simulink model "playback_data_4"  (R2015a)
settings: Solver=FixedStepDiscrete  SolverMode=SingleTasking  StartTime=0  StopTime=time_recorded(end)  FixedStep=sample_time  RelTol=1e-3
undefined symbols (not defined in the file): A1_notch_f1, A2_notch_f1, A_kalman_transverse, A_kalman_vertical, A_lpf_dtau, A_lpf_fourbar_angles, A_lpf_imu, A_lpf_lateral_angle, A_lpf_leg_spring, B1_lpf_dtau, B1_lpf_fourbar_angles, B1_lpf_imu, B1_lpf_lateral_angle, B1_lpf_leg_spring, B1_notch_f1, B2_lpf_dtau, B2_lpf_fourbar_angles, B2_lpf_imu, B2_lpf_lateral_angle, B2_lpf_leg_spring, B2_notch_f1, B_dx_versus_x0, B_kalman_transverse, B_kalman_vertical, backwards_K_front_of_t_row1, backwards_K_front_of_t_row2, backwards_K_sag_of_t, backwards_P_front_of_t, backwards_P_sag_of_t, C_kalman_transverse, C_kalman_vertical, com_leg_motor, com_torso, contact_threshold, control_start_time, d_ankle_to_foot, d_vertical_com, desired_com_forward_velocity, desired_com_lateral_velocity, desired_initial_leg_roll_left, desired_initial_leg_roll_right, desired_lateral_symmetry_angle, desired_standing_torso_pitch, desired_standing_torso_roll, desired_standing_z, desired_torso_pitch, desired_torso_roll, Discrete, fcut_contact, forward_dx_of_dxstar, forward_x_of_dxstar, g, gain_nodes_sea_torque, HIP_MTR_MAX_CONT_TORQUE, HIP_MTR_MAX_TORQUE, i_leg_motor, i_robot, i_torso, initial_dx_estimate, initial_dy_estimate ... (+75)
libraries: simulink x12, ctrlSharedLib x3
(part 1 of 5)
settings Model: CovSFcnEnable=off  Creator=wmartin  LastModifiedBy=wmartin
settings SolverCC: EnableConcurrentExecution=on
settings DataIOCC: LimitDataPoints=off  MaxDataPoints=1000000000  SaveFormat=StructureWithTime  SignalLogging=off  DSMLogging=off  VisualizeSimOutput=off
settings OptimizationCC: BlockReduction=off  OptimizeBlockIOStorage=off  BufferReuse=off  GlobalBufferReuse=off  ExpressionFolding=off  ExpressionDepthLimit=2147483647  LocalBlockOutputs=off  SimCompilerOptimization=on
settings DebuggingCC: UnderspecifiedInitializationDetection=Classic  MergeDetectMultiDrivingBlocksExec=none  SolverPrmCheckMsg=warning  StateNameClashWarn=warning
settings HardwareCC: ProdIntDivRoundTo=Zero  ProdEndianess=LittleEndian  ProdLongLongMode=on  ProdHWDeviceType=Generic->32-bit x86 compatible
settings ModelReferenceCC: UpdateModelReferenceTargets=IfOutOfDate  ModelReferenceNumInstancesAllowed=Single  ModelReferenceMinAlgLoopOccurrences=on
settings RTWCC: SystemTargetFile=slrt.tlc  TemplateMakefile=slrt_default_tmf  Description=Simulink Real-Time  RTWVerbose=off  RTWCompilerOptimization=on
settings CodeAppCC: MaxIdLength=256
settings SimulinkRealTimeCC: GeneratePreprocessorConditionals=Disable all

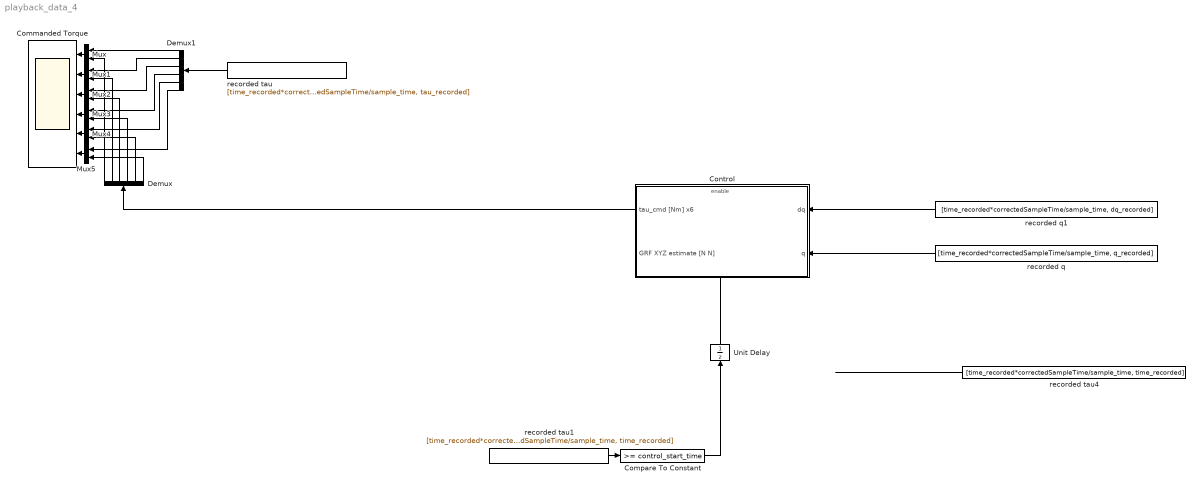
== system playback_data_4 ==
  Commanded Torque : Scope  NumInputPorts=6
      settings: TimeRange=75  YMin=-75~-150~31~-1~-1~12.5  YMax=125~50~44~1~1~37.5  SampleInput=on
  Compare To Constant : simulink/Logic and Bit Operations/Compare To Constant  relop=>=  const=control_start_time  OutDataTypeStr=boolean
  Control : Subsystem
  Demux : Demux  Outputs=6
  Demux1 : Demux  Outputs=6
  Mux{,1..5} (6 alike) : Mux  Inputs=2
  Unit Delay : UnitDelay  SampleTime=-1
  recorded q : FromWorkspace  VariableName=[time_recorded*correctedSampleTime/sample_time, q_recorded]  OutDataTypeStr=double  SampleTime=sample_time  OutputAfterFinalValue=Holding final value
  recorded q1 : FromWorkspace  VariableName=[time_recorded*correctedSampleTime/sample_time, dq_recorded]  OutDataTypeStr=double  SampleTime=sample_time  OutputAfterFinalValue=Holding final value
  recorded tau : FromWorkspace  VariableName=[time_recorded*correctedSampleTime/sample_time, tau_recorded]  OutDataTypeStr=double  SampleTime=sample_time  Interpolate=off  OutputAfterFinalValue=Holding final value
  recorded tau1 : FromWorkspace  VariableName=[time_recorded*correctedSampleTime/sample_time, time_recorded]  OutDataTypeStr=double  SampleTime=sample_time  OutputAfterFinalValue=Holding final value
  recorded tau4 : FromWorkspace  VariableName=[time_recorded*correctedSampleTime/sample_time, time_recorded]  OutDataTypeStr=double  SampleTime=sample_time  OutputAfterFinalValue=Holding final value
  wires:
  recorded tau1/1 -> Compare To Constant/1
  Unit Delay/1 -> Control/Enable
  recorded q1/1 -> Control/1(dq)
  recorded q/1 -> Control/2(q)
  Control/1(tau_cmd [Nm] x6) -> Demux/1
  recorded tau/1 -> Demux1/1
  Mux/1 -> Commanded Torque/1
  Mux1/1 -> Commanded Torque/2
  Mux2/1 -> Commanded Torque/3
  Mux3/1 -> Commanded Torque/4
  Mux4/1 -> Commanded Torque/5
  Mux5/1 -> Commanded Torque/6
  Demux1/1 -> Mux/1
  Demux/1 -> Mux/2
  Demux1/2 -> Mux1/1
  Demux1/3 -> Mux2/1
  Demux1/4 -> Mux3/1
  Demux1/5 -> Mux4/1
  Demux1/6 -> Mux5/1
  Demux/2 -> Mux1/2
  Demux/3 -> Mux2/2
  Demux/4 -> Mux3/2
  Demux/5 -> Mux4/2
  Demux/6 -> Mux5/2
  recorded tau4/1 -> ?
  Compare To Constant/1 -> Unit Delay/1

== system playback_data_4/Control ==
  dq : Inport
  q : Inport  Port=2
  Enable : EnablePort  StatesWhenEnabling=reset  PropagateVarSize=During execution
  Behavior Control : Subsystem
  Filter Velocities : Subsystem
  Subsystem : Subsystem
  tau_cmd [Nm] x6 : Outport  InitialOutput=[0 0 0 0 0 0]
  GRF XYZ estimate [N N] : Outport  Port=2  InitialOutput=[0 0 0]
  wires:
  dq/1 -> Filter Velocities/1(raw dq)
  Filter Velocities/1(filtered dq) -> Subsystem/5(dq), Behavior Control/1(dq)
  Behavior Control/4(GRF XYZ estimates [N N N]) -> GRF XYZ estimate [N N]/1
  q/1 -> Subsystem/4(q), Behavior Control/2(q)
  Behavior Control/1(Motor Torque Command [Nm] x6) -> Subsystem/1(Desired Torque [Nm] x6)
  Behavior Control/2(SEA Torque Velocity Command [Nm] x4) -> Subsystem/2(Desired SEA Torque Velocity [Nm] x4)
  Behavior Control/3(Force / Position Control [1/0] x4) -> Subsystem/3(Enable SEA Control [1/0] x4)
  Subsystem/1(tau_cmd [Nm] x6) -> tau_cmd [Nm] x6/1

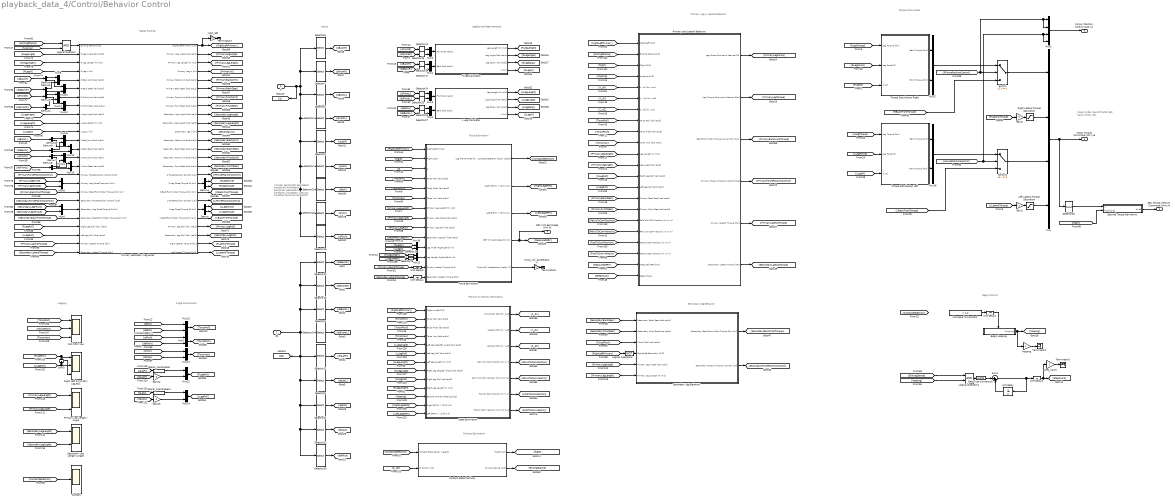
== system playback_data_4/Control/Behavior Control ==
  note: Logging
  note: Contact Estimation
  note: Angle Conversions
  note: Motor Order:
      |
      | backR
      | frontR
      | latR
      | backL
      | frontL
      | latL
  note: q Order:
      |
      | backJointR
      | backGearR
      | frontJointR
      | frontGearR
      |
      | backJointL
      | backGearL
      | frontJointL
      | frontGearL
      |
      | latR
      | latL
      |
      | torsoRoll
      | torsoYaw
      | torsoPitch
  note: Inputs
  note: Primary Leg + Lateral Behavior
  note: Secondary Leg Behavior
  note: Torque Commands
  note: Leg/Spring Measurements
  note: Force Estimation
  note: Position & Velocity Estimation
  note: Begin Control
  note: Signal Routing
  dq : Inport
  q : Inport  Port=2
  Begin Hopping : Subsystem
  Compare To Constant : simulink/Logic and Bit Operations/Compare To Constant  relop=>  const=1.2  OutDataTypeStr=boolean
  Contact : Scope
      settings: YMin=0.3  YMax=0.9  SaveName=ScopeData11  SampleInput=on
  Contact State Machine : Subsystem
  Data Type Conversion : DataTypeConversion  OutDataTypeStr=uint32
  Demux{,1,3..10} (10 alike) : Demux  Outputs=2
  Desired Torque Derivative : Subsystem
  Force Estimation : Subsystem
  Gain{1..2,12..13} (4 alike) : Gain  Gain=-1
  L Leg Calculator : Subsystem
  Left Lateral Torque Saturation : Saturate  UpperLimit=max_torque_lateral  LowerLimit=-max_torque_lateral
      settings: AttributesFormatString=Top: %<UpperLimit>\nBottom: %<LowerLimit>
  Logical Operator : Logic  IconShape=distinctive  AllPortsSameDT=off  OutDataTypeStr=boolean
  Logical Operator1 : Logic  AllPortsSameDT=off  OutDataTypeStr=boolean
  Logical Operator3 : Logic  Operator=NOT  AllPortsSameDT=off  OutDataTypeStr=boolean
  Mux : Mux
  Mux{1..2,4..24} (23 alike) : Mux  Inputs=2
  Mux3 : Mux
  Primary Leg Length / Angle : Scope  NumInputPorts=2
      settings: YMin=0.3~0  YMax=0.9~3.5  SaveName=ScopeData21  SampleInput=on
  Primary Secondary Leg Swap : Subsystem
  Primary and Lateral Behavior : Subsystem
  R Leg Calculator : Subsystem
  Right Lateral Torque Saturation : Saturate  UpperLimit=max_torque_lateral  LowerLimit=-max_torque_lateral
      settings: AttributesFormatString=Top: %<UpperLimit>\nBottom: %<LowerLimit>
  Right Left Symmetry Leg Roll : Scope  NumInputPorts=3
      settings: YMin=-0.2~-0.5~-0.5  YMax=1.3~1.8~0.5  SaveName=ScopeData19  SampleInput=on
  Roll Pitch Yaw : Scope  NumInputPorts=3
      settings: YMin=-1000~-5~-5  YMax=1000~5~5  SampleInput=on
  Secondary Leg Behavior : Subsystem
  Secondary Leg Length / Angle : Scope  NumInputPorts=2
      settings: YMin=-1~-0.8  YMax=1~1.4  SaveName=ScopeData22  SampleInput=on
  Selector1 : Selector  InputPortWidth=13  Indices=[10]
  Selector10 : Selector  InputPortWidth=13  Indices=[7 8]
  Selector11 : Selector  InputPortWidth=13  Indices=[9]
  Selector12 : Selector  InputPortWidth=13  Indices=[1 2]
  Selector13 : Selector  InputPortWidth=13  Indices=[3 4]
  Selector{14..17,19,24..27,29} (10 alike) : Selector  InputPortWidth=2  Indices=[1]
  Selector18 : Selector  InputPortWidth=13  Indices=[13]
  Selector2 : Selector  InputPortWidth=13  Indices=[5 6]
  Selector20 : Selector  InputPortWidth=13  Indices=[13]
  Selector21 : Selector  InputPortWidth=13  Indices=[11]
  Selector22 : Selector  InputPortWidth=13  Indices=[12]
  Selector23 : Selector  InputPortWidth=13  Indices=[11]
  Selector28 : Selector  InputPortWidth=13  Indices=[12]
  Selector33 : Selector  InputPortWidth=6  Indices=[1 2 4 5]
  Selector4 : Selector  InputPortWidth=13  Indices=[7 8]
  Selector5 : Selector  InputPortWidth=13  Indices=[9]
  Selector6 : Selector  InputPortWidth=13  Indices=[1 2]
  Selector7 : Selector  InputPortWidth=13  Indices=[3 4]
  Selector8 : Selector  InputPortWidth=13  Indices=[10]
  Selector9 : Selector  InputPortWidth=13  Indices=[5 6]
  State Estimation : Subsystem
  Sum1 : Sum  Inputs=|++  OutMin=0
  Sum3 : Sum  Inputs=-|+
  Switch : Switch  Criteria=u2 ~= 0
  Switch1 : Switch  Criteria=u2 ~= 0
  Terminator{1..3,6} (4 alike) : Terminator
  Torque Distribution Left : Subsystem
  Torque Distribution Right : Subsystem
  Unit Delay : UnitDelay  SampleTime=-1
  Unit Delay{1..4} (4 alike) : UnitDelay  SampleTime=sample_time
  hopping : Gain
  lateral_coordinates : Fcn  Expr=pi/2-u
  lateral_coordinates1 : Fcn  Expr=pi/2-u
  right_left : Gain
  step_count : Gain
  torso_roll_acceleration : Gain
  Motor Torque Command [Nm] x6 : Outport  OutputWhenDisabled=reset  InitialOutput=[0 0 0 0 0 0]
  SEA Torque Velocity Command [Nm] x4 : Outport  Port=2  OutputWhenDisabled=reset  InitialOutput=[0 0 0 0 0 0]
  Force / Position Control [1/0] x4 : Outport  Port=3  OutputWhenDisabled=reset  InitialOutput=[0 0 0 0 0 0]
  GRF XYZ estimates [N N N] : Outport  Port=4  OutputWhenDisabled=reset  InitialOutput=[0 0 0 0 0 0]
  wires:
  [dqYaw] -> Mux21/2
  [qYaw] -> Mux21/1
  [qPitch] -> Mux7/1
  [qRoll] -> Mux23/1
  dq/1 -> Selector9/1, Selector13/1, Selector12/1, Selector8/1, Selector22/1, Selector20/1, Selector21/1, Selector11/1, [dq], Selector10/1
  Selector21/1 -> [dqRoll]
  Selector22/1 -> [dqYaw]
  Selector20/1 -> [dqPitch]
  Selector10/1 -> [dqFrontL]
  Selector9/1 -> [dqBackL]
  Selector13/1 -> [dqFrontR]
  Selector12/1 -> [dqBackR]
  Selector11/1 -> [dqLatR]
  Selector8/1 -> [dqLatL]
  Gain12/1 -> Mux22/2
  Gain13/1 -> Mux24/2
  lateral_coordinates1/1 -> Mux24/1
  lateral_coordinates/1 -> Mux22/1
  Mux24/1 -> [LLegRoll]
  Mux22/1 -> [RLegRoll]
  [dqLatL] -> Gain13/1
  [qLatL] -> lateral_coordinates1/1
  [dqLatR] -> Gain12/1
  [qLatR] -> lateral_coordinates/1
  [dqPitch] -> Mux7/2
  [dqRoll] -> Mux23/2
  Mux7/1 -> [TorsoPitch]
  Mux23/1 -> [TorsoRoll]
  Mux21/1 -> [TorsoYaw]
  Secondary Leg Behavior/2(Secondary Force or Position Control [1/0]) -> [SecondaryForcePositionControl]
  Secondary Leg Behavior/1(Secondary Back/Front Motor Torque [Nm Nm]) -> [SecondaryBackFrontTorque]
  [ContactDetection] -> Contact/1
  [SecondaryLegAngle] -> Secondary Leg Length / Angle/2
  [SecondaryLegLength] -> Secondary Leg Length / Angle/1
  [PrimaryLegAngle] -> Primary Leg Length / Angle/2
  [PrimaryLegLength] -> Primary Leg Length / Angle/1
  Sum3/1 -> Right Left Symmetry Leg Roll/3
  [RLegRoll] -> Right Left Symmetry Leg Roll/1, Sum3/1
  [LLegRoll] -> Right Left Symmetry Leg Roll/2, Sum3/2
  [TorsoRoll] -> Roll Pitch Yaw/1
  [TorsoPitch] -> Roll Pitch Yaw/2
  [TorsoYaw] -> Roll Pitch Yaw/3
  [ExitingStance] -> Primary and Lateral Behavior/2(Exiting Stance [1/0])
  [Z_dZ] -> Contact State Machine/2("[Z dZ] [m m/s]")
  [ContactDetection] -> Contact State Machine/1(Contact Factor [body weight])
  [flight] -> Primary and Lateral Behavior/3(Flight [1/0])
  Contact State Machine/2(Exiting Stance [1/0]) -> [ExitingStance]
  [FootToComPosition] -> Primary and Lateral Behavior/19(Foot to COM Position [m m m])
  [FootToComVelocity] -> Primary and Lateral Behavior/20(Foot to COM Velocity [m m m])
  Contact State Machine/1(flight [1/0]) -> [flight]
  [PrimaryLegAngle] -> Primary and Lateral Behavior/12(Leg Angle [rad rad/s])
  [PrimaryBackGear] -> Primary and Lateral Behavior/15(Primary Back Gear [rad rad/s])
  [RightLeftPrimary] -> Primary and Lateral Behavior/1(Right/Left [1/0])
  [hopping] -> Primary and Lateral Behavior/4(Hopping [1/0])
  [PrimaryLegLength] -> Primary and Lateral Behavior/11(Leg Length [m m/s])
  [PrimaryFrontGear] -> Primary and Lateral Behavior/16(Primary Front Gear [rad rad/s])
  [TorsoPitch] -> Primary and Lateral Behavior/9(Torso Pitch [rad rad/s])
  [PelvisToComPosition] -> Primary and Lateral Behavior/17(Pelvis to COM Position [m m m])
  [PelvisToComVelocity] -> Primary and Lateral Behavior/18(Pelvis to COM Velocity [m m m])
  [X_dX] -> Primary and Lateral Behavior/5("[x, dx] [m, m/s]")
  [Z_dZ] -> Primary and Lateral Behavior/7("[z, dz] [m, m/s]")
  [TorsoRoll] -> Primary and Lateral Behavior/8(Torso Roll [rad rad/s])
  [MeasuredGRF] -> Primary and Lateral Behavior/21(Measured GRF [N N])
  [StepCount] -> Primary and Lateral Behavior/22(Steps Taken)
  [Y_dY] -> Primary and Lateral Behavior/6("[y,  dy] [m, m/s]")
  [RLegRoll] -> Primary and Lateral Behavior/13(Right Leg Roll [rad rad/s])
  [LLegRoll] -> Primary and Lateral Behavior/14(Left Leg Roll [rad rad/s])
  [TorsoYaw] -> Primary and Lateral Behavior/10(Torso Yaw [rad rad/s])
  State Estimation/7(Foot to COM Velocity [m/s m/s m/s]) -> [FootToComVelocity]
  State Estimation/6(Foot to COM Position [m m m]) -> [FootToComPosition]
  [flight] -> Desired Torque Derivative/2(flight [1/0])
  Gain1/1 -> Left Lateral Torque Saturation/1
  Gain2/1 -> Right Lateral Torque Saturation/1
  Begin Hopping/1(Hopping?) -> hopping/1, [hopping]
  Unit Delay4/1 -> Force Estimation/14(Secondary Lateral Torque [Nm])
  Unit Delay3/1 -> Force Estimation/13(Primary Lateral Torque [Nm])
  Selector29/1 -> Mux20/2
  [LLegLength] -> Selector29/1
  Selector19/1 -> Mux20/1
  Primary and Lateral Behavior/5(Primary Lateral Torque [Nm]) -> [PrimaryLateralTorque]
  Primary and Lateral Behavior/6(Secondary Lateral Torque [Nm]) -> [SecondaryLateralTorque]
  Left Lateral Torque Saturation/1 -> Mux/4
  Right Lateral Torque Saturation/1 -> Mux/2
  Primary Secondary Leg Swap/25(Left Lateral Torque [Nm]) -> [LLateralTorque]
  Primary Secondary Leg Swap/24(Right Lateral Torque [Nm]) -> [RLateralTorque]
  [SecondaryLateralTorque] -> Primary Secondary Leg Swap/25(Secondary Lateral Torque [Nm])
  [PrimaryLateralTorque] -> Primary Secondary Leg Swap/24(Primary Lateral Torque [Nm])
  Force Estimation/5(Torso Roll Acceleration [rad/s^2]) -> torso_roll_acceleration/1
  torso_roll_acceleration/1 -> Terminator6/1
  [SecondaryLateralTorque] -> Unit Delay4/1
  [PrimaryLateralTorque] -> Unit Delay3/1
  [SecondaryLegRoll] -> Force Estimation/10(Secondary Leg Roll [rad rad/s])
  Mux20/1 -> Force Estimation/12(Leg Length Right/Left [m m])
  [RLegLength] -> Selector19/1
  Mux19/1 -> Force Estimation/11(Leg Width Right/Left [m m])
  [LLegW] -> Mux19/2
  [RLegW] -> Mux19/1
  [PrimaryLegRoll] -> Force Estimation/9(Primary Leg Roll [rad rad/s])
  [PrimaryLegAngle] -> Force Estimation/8(Primary Leg Angle [rad rad/s])
  [PrimaryLegLength] -> Force Estimation/7(Primary Leg Length [m m/s])
  [q] -> Force Estimation/3(q)
  [TorsoPitch] -> Force Estimation/5(Torso Pitch [rad rad/s])
  [TorsoYaw] -> Force Estimation/6(Torso Yaw [rad rad/s])
  [TorsoRoll] -> Force Estimation/4(Torso Roll [rad rad/s])
  [flight] -> Force Estimation/2(Flight [1/0])
  [RightLeftPrimary] -> Force Estimation/1(Right/Left Primary)
  [TorsoYaw] -> State Estimation/4(Torso Yaw [rad rad/s])
  [ExitingStance] -> Logical Operator/1
  [hopping] -> Logical Operator/2
  [hopping] -> Logical Operator1/2
  [ExitingStance] -> Logical Operator1/1
  State Estimation/2("Lateral COM [m, m/s]") -> [Y_dY]
  Unit Delay2/1 -> [StepCount], step_count/1
  step_count/1 -> Terminator3/1
  State Estimation/5(Pelvis to COM Velocity [m/s m/s m/s]) -> [PelvisToComVelocity]
  State Estimation/4(Pelvis to COM Position [m m m]) -> [PelvisToComPosition]
  [LLegRoll] -> Primary Secondary Leg Swap/23("Left Leg Roll [rad, rad/s]")
  [RLegRoll] -> Primary Secondary Leg Swap/22("Right Leg Roll [rad, rad/s]")
  Primary Secondary Leg Swap/23("Secondary Leg Roll [rad, rad/s]") -> [SecondaryLegRoll]
  Primary Secondary Leg Swap/22("Primary Leg Roll [rad, rad/s]") -> [PrimaryLegRoll]
  Force Estimation/4(GRF XYZ estimates [N N N]) -> [MeasuredGRF], GRF XYZ estimates [N N N]/1
  [RLegForce] -> Torque Distribution Right/2(Leg Force [N])
  [LLegForce] -> Torque Distribution Left/2(Leg Force [N])
  Force Estimation/3(Left GRF [X Y Z] [N N N]) -> [LeftLegGRFs]
  [LLateralTorque] -> Gain1/1
  [LeftLegGRFs] -> State Estimation/13(Left GRF [X Y Z] [N N N])
  [RightLegGRFs] -> State Estimation/12(Right GRF [X Y Z] [N N N])
  Force Estimation/2(Right GRF [X Y Z] [N N N]) -> [RightLegGRFs]
  [hopping] -> State Estimation/11(Enable Kalman Filtering [1/0])
  [RightLeftPrimary] -> State Estimation/1(Right or Left [1/0])
  [RLegAngle] -> State Estimation/8(Right Leg Sagittal Angle [rad rad/s])
  [LLegAngle] -> State Estimation/5(Left Leg Sagittal Angle [rad rad/s])
  [LLegLength] -> State Estimation/7(Left Leg Length [m m/s])
  [LLegRoll] -> State Estimation/6(Left Leg Roll [rad rad/s])
  [RLegRoll] -> State Estimation/9(Right Leg Roll [rad rad/s])
  [TorsoPitch] -> State Estimation/3(Torso Pitch [rad rad/s])
  [TorsoRoll] -> State Estimation/2(Torso Roll [rad rad/s])
  [RLegLength] -> State Estimation/10(Right Leg Length [m m/s])
  State Estimation/3("Vertical COM [m, m/s]") -> [Z_dZ]
  State Estimation/1("Horizontal COM [m, m/s]") -> [X_dX]
  Force Estimation/1(Leg Plane Force for Contact Detection [body weight]) -> [ContactDetection]
  Selector28/1 -> [qYaw]
  [PrimaryLegLength] -> Secondary Leg Behavior/6(Primary Leg Length [m m/s])
  Mux/1 -> Motor Torque Command [Nm] x6/1, Selector33/1
  Desired Torque Derivative/1(dx/dt) -> SEA Torque Velocity Command [Nm] x4/1
  Selector33/1 -> Desired Torque Derivative/1(x)
  [PrimaryLegAngle] -> Secondary Leg Behavior/5(Primary Leg Angle [rad rad/s])
  Selector4/1 -> [qFrontL]
  Selector2/1 -> [qBackL]
  Selector7/1 -> [qFrontR]
  Selector6/1 -> [qBackR]
  Selector1/1 -> [qLatL]
  Selector5/1 -> [qLatR]
  [qBackR] -> Selector16/1
  [dqBackR] -> Selector17/1
  [qFrontR] -> Selector14/1
  [dqFrontR] -> Selector15/1
  Mux2/1 -> R Leg Calculator/1(Front [rad rad/s])
  Mux1/1 -> R Leg Calculator/2(Back [rad rad/s])
  R Leg Calculator/1("Leg Length [m m/s] ") -> [RLegLength]
  R Leg Calculator/2(Leg Angle [rad rad/s]) -> [RLegAngle]
  R Leg Calculator/3(Leg Splay [rad rad/s]) -> [RLegSplay]
  [RLegW] -> Torque Distribution Right/3(w [m])
  Selector14/1 -> Mux2/1
  Selector15/1 -> Mux2/2
  Selector17/1 -> Mux1/2
  Selector16/1 -> Mux1/1
  q/1 -> Selector6/1, Selector7/1, Selector2/1, Selector4/1, Selector5/1, Selector18/1, Selector28/1, Selector23/1, Selector1/1, [q]
  Selector18/1 -> [qPitch]
  [RLegTorque] -> Torque Distribution Right/1(Leg Torque [Nm])
  Selector23/1 -> [qRoll]
  [qBackL] -> Selector26/1
  [dqBackL] -> Selector27/1
  [qFrontL] -> Selector24/1
  [dqFrontL] -> Selector25/1
  Mux5/1 -> L Leg Calculator/1(Front [rad rad/s])
  Mux4/1 -> L Leg Calculator/2(Back [rad rad/s])
  L Leg Calculator/1("Leg Length [m m/s] ") -> [LLegLength]
  L Leg Calculator/2(Leg Angle [rad rad/s]) -> [LLegAngle]
  L Leg Calculator/3(Leg Splay [rad rad/s]) -> [LLegSplay]
  Selector24/1 -> Mux5/1
  Selector25/1 -> Mux5/2
  Selector27/1 -> Mux4/2
  Selector26/1 -> Mux4/1
  R Leg Calculator/4(w [m]) -> [RLegW]
  L Leg Calculator/4(w [m]) -> [LLegW]
  Primary and Lateral Behavior/1(Leg Force Command (stance) [N]) -> [PrimaryLegForce]
  Primary and Lateral Behavior/2(Leg Torque Command (stance) [Nm]) -> [PrimaryLegTorque]
  hopping/1 -> Terminator1/1
  [LLegTorque] -> Torque Distribution Left/1(Leg Torque [Nm])
  [LLegW] -> Torque Distribution Left/3(w [m])
  right_left/1 -> Terminator2/1
  Compare To Constant/1 -> Unit Delay1/1
  [TorsoPitch] -> Secondary Leg Behavior/3(Torso Pitch [rad rad/s])
  Mux3/1 -> Force / Position Control [1/0] x4/1
  Primary Secondary Leg Swap/2(Primary Leg Angle [rad rad/s]) -> [PrimaryLegAngle]
  Primary Secondary Leg Swap/4(Primary Leg w [m]) -> [PrimaryW]
  Primary Secondary Leg Swap/3(Primary Leg Length [m m/s]) -> [PrimaryLegLength]
  [RLegAngle] -> Primary Secondary Leg Swap/2(R Leg Angle [rad rad/s])
  [RLegLength] -> Primary Secondary Leg Swap/3(R Leg Length [m m/s])
  [RLegW] -> Primary Secondary Leg Swap/4(R Leg w [m])
  [LLegAngle] -> Primary Secondary Leg Swap/9(L Leg Angle [rad rad/s])
  [LLegLength] -> Primary Secondary Leg Swap/10(L Leg Length [m m/s])
  [LLegW] -> Primary Secondary Leg Swap/11(L Leg w [m])
  [SecondaryLegForce] -> Mux6/1
  [SecondaryLegTorque] -> Mux6/2
  Mux6/1 -> Primary Secondary Leg Swap/20(Secondary Leg Force/Torque [N Nm])
  Mux8/1 -> Primary Secondary Leg Swap/17(Primary Leg Force/Torque [N Nm])
  [PrimaryLegTorque] -> Mux8/2
  [PrimaryLegForce] -> Mux8/1
  Primary Secondary Leg Swap/10(Secondary Leg Length [rad rad/s]) -> [SecondaryLegLength]
  Primary Secondary Leg Swap/9(Secondary Leg Angle [rad rad/s]) -> [SecondaryLegAngle]
  Primary Secondary Leg Swap/20(L Leg Force/Torque [N Nm]) -> Demux/1
  Demux/1 -> [LLegForce]
  Demux/2 -> [LLegTorque]
  Primary Secondary Leg Swap/17(R Leg Force/Torque [N Nm]) -> Demux1/1
  Demux1/1 -> [RLegForce]
  Demux1/2 -> [RLegTorque]
  [qFrontR] -> Demux3/1
  [dqFrontR] -> Demux4/1
  Mux9/1 -> Primary Secondary Leg Swap/5(R Back Joint [rad rad/s])
  Mux10/1 -> Primary Secondary Leg Swap/6(R Back Gear [rad rad/s])
  Mux11/1 -> Primary Secondary Leg Swap/7(R Front Joint [rad rad/s])
  Mux12/1 -> Primary Secondary Leg Swap/8(R Front Gear [rad rad/s])
  Demux3/1 -> Mux11/1
  Demux3/2 -> Mux12/1
  Demux4/1 -> Mux11/2
  Demux4/2 -> Mux12/2
  [dqBackR] -> Demux5/1
  [qBackR] -> Demux6/1
  Demux6/1 -> Mux9/1
  Demux6/2 -> Mux10/1
  Demux5/1 -> Mux9/2
  Demux5/2 -> Mux10/2
  [qFrontL] -> Demux7/1
  [dqFrontL] -> Demux8/1
  Mux16/1 -> Primary Secondary Leg Swap/12(L Back Joint [rad rad/s])
  Mux13/1 -> Primary Secondary Leg Swap/13(L Back Gear [rad rad/s])
  Mux14/1 -> Primary Secondary Leg Swap/14(L Front Joint [rad rad/s])
  Mux15/1 -> Primary Secondary Leg Swap/15(L Front Gear [rad rad/s])
  Demux7/1 -> Mux14/1
  Demux7/2 -> Mux15/1
  Demux8/1 -> Mux14/2
  Demux8/2 -> Mux15/2
  [dqBackL] -> Demux9/1
  [qBackL] -> Demux10/1
  Demux10/1 -> Mux16/1
  Demux10/2 -> Mux13/1
  Demux9/1 -> Mux16/2
  Demux9/2 -> Mux13/2
  [PrimaryForcePositionControl] -> Primary Secondary Leg Swap/16(Primary Force/Position Control [1/0])
  [SecondaryForcePositionControl] -> Primary Secondary Leg Swap/19(Secondary Force/Position Control [1/0])
  [PrimaryBackFrontTorque] -> Primary Secondary Leg Swap/18(Primary Back/Front Motor Torque [Nm Nm])
  [SecondaryBackFrontTorque] -> Primary Secondary Leg Swap/21(Secondary Back/Front Motor Torque [Nm Nm])
  Primary Secondary Leg Swap/5(Primary Back Joint [rad rad/s]) -> [PrimaryBackJoint]
  Primary Secondary Leg Swap/6(Primary Back Gear [rad rad/s]) -> [PrimaryBackGear]
  Primary Secondary Leg Swap/7(Primary Front Joint [rad rad/s]) -> [PrimaryFrontJoint]
  Primary Secondary Leg Swap/8(Primary Front Gear [rad rad/s]) -> [PrimaryFrontGear]
  Primary Secondary Leg Swap/12(Secondary Back Joint [rad rad/s]) -> [SecondaryBackJoint]
  Primary Secondary Leg Swap/13(Secondary Back Gear [rad rad/s]) -> [SecondaryBackGear]
  Primary Secondary Leg Swap/14(Secondary Front Joint [rad rad/s]) -> [SecondaryFrontJoint]
  Primary Secondary Leg Swap/15(Secondary Front Gear [rad rad/s]) -> [SecondaryFrontGear]
  Primary Secondary Leg Swap/11(Secondary Leg w [m]) -> [SecondaryW]
  Primary Secondary Leg Swap/19(L Force/Position Control [1/0]) -> [LForcePositionControl]
  Primary Secondary Leg Swap/16(R Force/Position Control [1/0]) -> [RForcePositionControl]
  Primary Secondary Leg Swap/18(R Back/Front Motor Torque [Nm Nm]) -> [RBackFrontTorque]
  Primary Secondary Leg Swap/21(L Back/Front Motor Torque [Nm Nm]) -> [LBackFrontTorque]
  Logical Operator/1 -> Primary Secondary Leg Swap/1(Exiting Stance [1/0])
  Primary Secondary Leg Swap/1(Right/Left Primary [1/0]) -> [RightLeftPrimary], right_left/1
  Primary and Lateral Behavior/3(Back/Front Motor Torque (swing) [Nm Nm]) -> [PrimaryBackFrontTorque]
  Primary and Lateral Behavior/4(Primary Force or Position Control [1/0]) -> [PrimaryForcePositionControl]
  [RightLeftPrimary] -> Logical Operator3/1
  Logical Operator3/1 -> Secondary Leg Behavior/4(Right/Left Secondary [1/0])
  [SecondaryFrontGear] -> Secondary Leg Behavior/2(Secondary Front Gear [rad rad/s])
  [SecondaryBackGear] -> Secondary Leg Behavior/1(Secondary Back Gear [rad rad/s])
  [RForcePositionControl] -> Mux3/2, Mux3/1, Switch/2
  [LForcePositionControl] -> Mux3/4, Mux3/3, Switch1/2
  Switch/1 -> Mux/1
  [RLateralTorque] -> Gain2/1
  Torque Distribution Right/2(Front Torque [Nm]) -> Mux17/2
  Torque Distribution Right/1(Back Torque [Nm]) -> Mux17/1
  Torque Distribution Left/1(Back Torque [Nm]) -> Mux18/1
  Torque Distribution Left/2(Front Torque [Nm]) -> Mux18/2
  Mux17/1 -> Switch/1
  [RBackFrontTorque] -> Switch/3
  Mux18/1 -> Switch1/1
  [LBackFrontTorque] -> Switch1/3
  Switch1/1 -> Mux/3
  Unit Delay/1 -> Sum1/2
  Sum1/1 -> Unit Delay2/1, Unit Delay/1
  Logical Operator1/1 -> Data Type Conversion/1
  Data Type Conversion/1 -> Sum1/1
  Unit Delay1/1 -> Begin Hopping/Enable

== system playback_data_4/Control/Filter Velocities ==
  raw dq : Inport
  Demux : Demux  Outputs=3
  Demux1 : Demux  Outputs=3
  Demux2 : Demux  Outputs=2
  Demux3 : Demux  Outputs=2
  Fourbar : Selector  InputPortWidth=13  Indices=[1 2 3 4 5 6 7 8]
  Fourbar Velocity Filter : Scope  NumInputPorts=4
      settings: YMin=-0.55~-0.4~-0.4~-0.6  YMax=0.25~0.7~0.45~0.5  SaveName=ScopeData14  SampleInput=on
  IMU Two Pole Filter : DiscreteTransferFcn  Numerator=[A_lpf_imu 0 0]  Denominator=[1 B1_lpf_imu B2_lpf_imu]  SampleTime=sample_time
  Lateral : Selector  InputPortWidth=13  Indices=[9 10]
  Lateral Angle Two Pole Filter1 : DiscreteTransferFcn  Numerator=[A_lpf_lateral_angle 0 0]  Denominator=[1 B1_lpf_lateral_angle B2_lpf_lateral_angle]  SampleTime=sample_time
  Lateral Angle Two Pole Filter2 : DiscreteTransferFcn  Numerator=[A_lpf_fourbar_angles 0 0]  Denominator=[1 B1_lpf_fourbar_angles B2_lpf_fourbar_angles]  SampleTime=sample_time
  Leg Roll Velocity Filter : Scope  NumInputPorts=2
      settings: YMin=-0.225~-1.5  YMax=0.175~2.25  SaveName=LegRollFilter  SampleInput=on
  Mux : Mux  Inputs=3
  Mux{25..33} (9 alike) : Mux  Inputs=2
  Selector1 : Selector  InputPortWidth=8  Indices=[1 2]
  Selector2 : Selector  InputPortWidth=8  Indices=[3 4]
  Selector3 : Selector  InputPortWidth=8  Indices=[5 6]
  Selector34 : Selector  InputPortWidth=8  Indices=[1 2]
  Selector35 : Selector  InputPortWidth=8  Indices=[3 4]
  Selector36 : Selector  InputPortWidth=8  Indices=[5 6]
  Selector37 : Selector  InputPortWidth=8  Indices=[7 8]
  Selector4 : Selector  InputPortWidth=8  Indices=[7 8]
  Torso Orientation : Selector  InputPortWidth=13  Indices=[11 12 13]
  Torso Orientation Filter : Scope  NumInputPorts=3
      settings: YMin=-0.2~-0.03~-0.15  YMax=0.125~0.0275~0.15  SaveName=ScopeData13  SampleInput=on
  filtered dq : Outport
  wires:
  Selector1/1 -> Mux30/2
  Selector2/1 -> Mux31/2
  Selector3/1 -> Mux32/2
  Selector4/1 -> Mux33/2
  Demux3/2 -> Mux29/2
  Demux3/1 -> Mux28/2
  Demux2/1 -> Mux28/1
  Demux2/2 -> Mux29/1
  Demux1/3 -> Mux27/2
  Demux1/2 -> Mux26/2
  Demux1/1 -> Mux25/2
  Demux/3 -> Mux27/1
  Demux/2 -> Mux26/1
  Demux/1 -> Mux25/1
  Mux29/1 -> Leg Roll Velocity Filter/2
  Mux28/1 -> Leg Roll Velocity Filter/1
  Selector37/1 -> Mux33/1
  Selector36/1 -> Mux32/1
  Selector35/1 -> Mux31/1
  Fourbar/1 -> Lateral Angle Two Pole Filter2/1, Selector37/1, Selector36/1, Selector35/1, Selector34/1
  Selector34/1 -> Mux30/1
  Mux33/1 -> Fourbar Velocity Filter/4
  Mux31/1 -> Fourbar Velocity Filter/2
  Mux32/1 -> Fourbar Velocity Filter/3
  Mux30/1 -> Fourbar Velocity Filter/1
  Mux26/1 -> Torso Orientation Filter/2
  Mux27/1 -> Torso Orientation Filter/3
  Mux25/1 -> Torso Orientation Filter/1
  Lateral Angle Two Pole Filter1/1 -> Mux/2, Demux3/1
  Torso Orientation/1 -> Demux/1, IMU Two Pole Filter/1
  Lateral/1 -> Lateral Angle Two Pole Filter1/1, Demux2/1
  raw dq/1 -> Lateral/1, Torso Orientation/1, Fourbar/1
  Mux/1 -> filtered dq/1
  IMU Two Pole Filter/1 -> Mux/3, Demux1/1
  Lateral Angle Two Pole Filter2/1 -> Mux/1, Selector1/1, Selector2/1, Selector3/1, Selector4/1

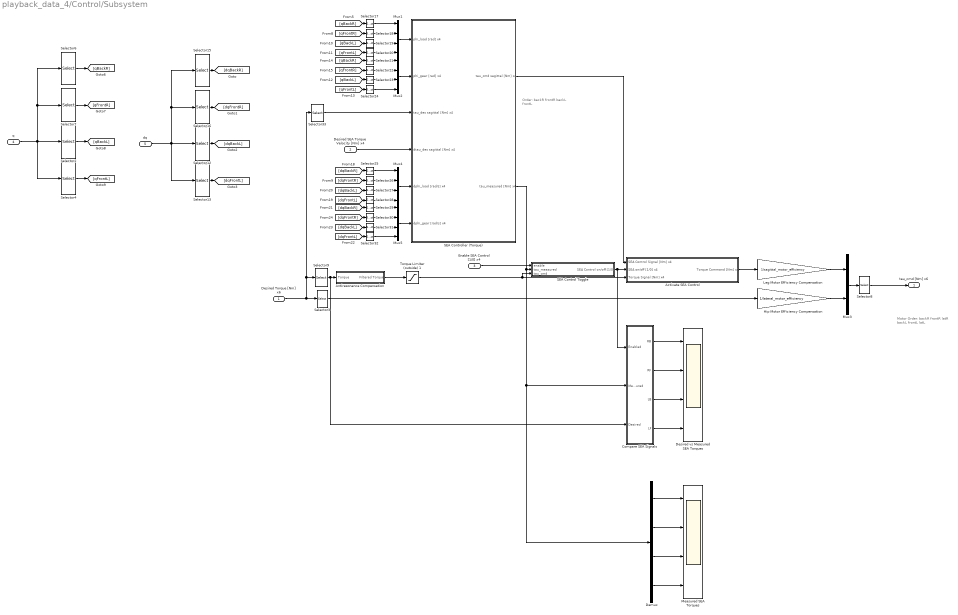
== system playback_data_4/Control/Subsystem ==
  note: Order:
      | backR
      | frontR
      | backL
      | frontL
  note: Motor Order:
      |
      | backR
      | frontR
      | latR
      | backL
      | frontL
      | latL
  Desired Torque [Nm] x6 : Inport  OutDataTypeStr=double  PortDimensions=6  SampleTime=sample_time
  Desired SEA Torque Velocity [Nm] x4 : Inport  Port=2  OutDataTypeStr=double  PortDimensions=4  SampleTime=sample_time
  Enable SEA Control [1/0] x4 : Inport  Port=3  OutDataTypeStr=boolean  PortDimensions=4  SampleTime=sample_time
  q : Inport  Port=4  OutDataTypeStr=double  PortDimensions=13  SampleTime=sample_time
  dq : Inport  Port=5  OutDataTypeStr=double  PortDimensions=13  SampleTime=sample_time
  Activate SEA Control : Subsystem
  Antiresonance Compensation : Subsystem
  Compare SEA Signals : Subsystem
  Demux : Demux
  Desired vs Measured SEA Torques : Scope  NumInputPorts=4
      settings: YMin=-1000~-5~-5~-5  YMax=1000~5~5~5  SampleInput=on
  Hip Motor Efficiency Compensation : Gain  Gain=1/lateral_motor_efficiency
  Leg Motor Efficiency Compensation : Gain  Gain=1/sagittal_motor_efficiency
  Measured SEA Torques : Scope  NumInputPorts=4
      settings: YMin=-200~-350~-300~-150  YMax=50~50~50~200  SampleInput=on
  Mux{1..2,4..5} (4 alike) : Mux
  Mux3 : Mux  Inputs=2
  SEA Control Toggle : Subsystem
  SEA Controller (Torque) : Subsystem
  Selector12 : Selector  InputPortWidth=13  Indices=[5 6]
  Selector13 : Selector  InputPortWidth=13  Indices=[7 8]
  Selector15 : Selector  InputPortWidth=13  Indices=[1 2]
  Selector16 : Selector  InputPortWidth=13  Indices=[3 4]
  Selector{17..20,25..28} (8 alike) : Selector  InputPortWidth=2  Indices=[1]
  Selector2 : Selector  InputPortWidth=13  Indices=[5 6]
  Selector{21..24,29..32} (8 alike) : Selector  InputPortWidth=2  Indices=[2]
  Selector3 : Selector  InputPortWidth=6  Indices=[3 6]
  Selector33 : Selector  InputPortWidth=6  Indices=[1 2 4 5]
  Selector4 : Selector  InputPortWidth=13  Indices=[7 8]
  Selector6 : Selector  InputPortWidth=13  Indices=[1 2]
  Selector7 : Selector  InputPortWidth=13  Indices=[3 4]
  Selector8 : Selector  InputPortWidth=6  Indices=[1 2 5 3 4 6]
  Selector9 : Selector  InputPortWidth=6  Indices=[1 2 4 5]
  Torque Limiter (outside) 1 : Saturate  UpperLimit=max_sagittal_unloaded_torque  LowerLimit=-max_sagittal_unloaded_torque
      settings: AttributesFormatString=Hi: %<UpperLimit>\nLo: %<LowerLimit>
  tau_cmd [Nm] x6 : Outport  OutDataTypeStr=double  PortDimensions=6  SampleTime=0  InitialOutput=[0 0 0 0 0 0]
  wires:
  Torque Limiter (outside) 1/1 -> Activate SEA Control/3(Torque Signal [Nm] x4), SEA Control Toggle/3(tau_cmd)
  Selector9/1 -> Compare SEA Signals/3(Desired), Antiresonance Compensation/1(Torque)
  SEA Controller (Torque)/2(tau_measured [Nm] x4) -> Demux/1, Compare SEA Signals/2(Measured), SEA Control Toggle/2(tau_measured)
  SEA Controller (Torque)/1(tau_cmd sagittal [Nm] x4) -> Activate SEA Control/1(SEA Control Signal [Nm] x4)
  Enable SEA Control [1/0] x4/1 -> SEA Control Toggle/1(enable)
  Activate SEA Control/1(Torque Command [Nm] x4) -> Leg Motor Efficiency Compensation/1
  Demux/4 -> Measured SEA Torques/4
  Demux/1 -> Measured SEA Torques/1
  SEA Control Toggle/1(SEA Control on/off [1/0]) -> Compare SEA Signals/1(Enabled), Activate SEA Control/2("SEA on/off [1/0] x4 ")
  Leg Motor Efficiency Compensation/1 -> Mux3/1
  Hip Motor Efficiency Compensation/1 -> Mux3/2
  Compare SEA Signals/2(RF) -> Desired vs Measured SEA Torques/2
  Demux/3 -> Measured SEA Torques/3
  Demux/2 -> Measured SEA Torques/2
  Compare SEA Signals/4(LF) -> Desired vs Measured SEA Torques/4
  Compare SEA Signals/3(LB) -> Desired vs Measured SEA Torques/3
  Antiresonance Compensation/1(Filtered Torque) -> Torque Limiter (outside) 1/1
  Desired SEA Torque Velocity [Nm] x4/1 -> SEA Controller (Torque)/4(dtau_des sagittal [Nm] x4)
  Compare SEA Signals/1(RB) -> Desired vs Measured SEA Torques/1
  Selector26/1 -> Mux4/2
  [dqBackR] -> Selector29/1
  Selector28/1 -> Mux4/4
  Selector25/1 -> Mux4/1
  Selector3/1 -> Hip Motor Efficiency Compensation/1
  [dqFrontL] -> Selector32/1
  Selector32/1 -> Mux5/4
  Mux3/1 -> Selector8/1
  [dqFrontR] -> Selector30/1
  [dqBackL] -> Selector31/1
  Selector33/1 -> SEA Controller (Torque)/3(tau_des sagittal [Nm] x4)
  [dqBackL] -> Selector27/1
  Selector31/1 -> Mux5/3
  Selector29/1 -> Mux5/1
  Mux5/1 -> SEA Controller (Torque)/6(dphi_gear [rad/s] x4)
  [dqFrontL] -> Selector28/1
  Selector30/1 -> Mux5/2
  [dqBackR] -> Selector25/1
  Selector27/1 -> Mux4/3
  [dqFrontR] -> Selector26/1
  Mux4/1 -> SEA Controller (Torque)/5(dphi_load [rad/s] x4)
  [qBackR] -> Selector17/1
  [qBackL] -> Selector19/1
  Selector17/1 -> Mux1/1
  Selector13/1 -> [dqFrontL]
  [qBackL] -> Selector23/1
  Selector24/1 -> Mux2/4
  Selector21/1 -> Mux2/1
  [qFrontL] -> Selector24/1
  Selector23/1 -> Mux2/3
  Selector22/1 -> Mux2/2
  [qFrontR] -> Selector22/1
  Selector18/1 -> Mux1/2
  Mux2/1 -> SEA Controller (Torque)/2(phi_gear [rad] x4)
  [qFrontL] -> Selector20/1
  [qFrontR] -> Selector18/1
  Selector20/1 -> Mux1/4
  Selector16/1 -> [dqFrontR]
  [qBackR] -> Selector21/1
  Selector12/1 -> [dqBackL]
  Mux1/1 -> SEA Controller (Torque)/1(phi_load [rad] x4)
  Selector19/1 -> Mux1/3
  dq/1 -> Selector13/1, Selector15/1, Selector16/1, Selector12/1
  Selector4/1 -> [qFrontL]
  Selector6/1 -> [qBackR]
  Selector15/1 -> [dqBackR]
  Selector7/1 -> [qFrontR]
  Selector2/1 -> [qBackL]
  q/1 -> Selector2/1, Selector7/1, Selector6/1, Selector4/1
  Selector8/1 -> tau_cmd [Nm] x6/1
  Desired Torque [Nm] x6/1 -> Selector33/1, Selector9/1, Selector3/1

== system playback_data_4/Control/Behavior Control/Begin Hopping ==
  Enable : EnablePort  StatesWhenEnabling=reset
  Constant : Constant
  Hopping? : Outport  InitialOutput=[0]
  wires:
  Constant/1 -> Hopping?/1

== system playback_data_4/Control/Behavior Control/Contact State Machine ==
  Contact Factor [body weight] : Inport
  "[Z dZ] [m m/s]" : Inport  Port=2
  Detect Fall Nonpositive : simulink/Logic and Bit Operations/Detect Fall Nonpositive  vinit=0  InputProcessing=Inherited  OutDataTypeStr=boolean
  Mux25 : Mux  Inputs=5
  Selector : Selector  InputPortWidth=2  Indices=[2]
  State Machine : State Transition Table  TreatAsAtomicUnit=on
  Terminator8 : Terminator
  Unit Delay5 : UnitDelay  SampleTime=-1
  Unit Delay6 : UnitDelay  SampleTime=sample_time
  Unit Delay7 : UnitDelay  SampleTime=sample_time
  Unit Delay8 : UnitDelay  SampleTime=sample_time
  flight [1/0] : Outport
  Exiting Stance [1/0] : Outport  Port=2
  wires:
  "[Z dZ] [m m/s]"/1 -> Selector/1
  State Machine/1(" TouchDown") -> Mux25/1
  State Machine/2(" LockedContact") -> Mux25/2
  State Machine/3(" Unloading") -> Mux25/3
  Mux25/1 -> Unit Delay8/1
  State Machine/5(" Flight") -> Unit Delay7/1, Mux25/5
  Unit Delay5/1 -> State Machine/2(previous_z_velocity)
  Contact Factor [body weight]/1 -> State Machine/3(vertical_grf)
  Selector/1 -> Unit Delay5/1, State Machine/1(z_velocity)
  Unit Delay8/1 -> Terminator8/1
  State Machine/4(" Takeoff") -> Mux25/4, Unit Delay6/1
  Unit Delay6/1 -> Detect Fall Nonpositive/1
  Unit Delay7/1 -> flight [1/0]/1
  Detect Fall Nonpositive/1 -> Exiting Stance [1/0]/1

== system playback_data_4/Control/Behavior Control/Desired Torque Derivative ==
  x : Inport
  flight [1/0] : Inport  Port=2
  Detect Change : simulink/Logic and Bit Operations/Detect Change  vinit=0  InputProcessing=Inherited  OutDataTypeStr=boolean
  Gain1 : Gain  Gain=1/sample_time
  Logical Operator : Logic  Operator=NOT  AllPortsSameDT=off  OutDataTypeStr=boolean
  Product : Product
  difference : simulink/Discrete/Difference  ICPrevInput=0.0  InputProcessing=Inherited  OutMin=[]  OutMax=[]  OutDataType=fixdt(1, 16)  OutScaling=2^-10  DoSatur=off
  two_pole_filter : DiscreteTransferFcn  Numerator=[A_lpf_dtau 0 0]  Denominator=[1 B1_lpf_dtau B2_lpf_dtau]  ExternalReset=Either  SampleTime=sample_time
      settings: InputPortMap=u0,r7
  dx/dt : Outport
  wires:
  Gain1/1 -> difference/1
  x/1 -> Gain1/1
  two_pole_filter/1 -> dx/dt/1
  flight [1/0]/1 -> two_pole_filter/2, Detect Change/1
  difference/1 -> Product/1
  Product/1 -> two_pole_filter/1
  Detect Change/1 -> Logical Operator/1
  Logical Operator/1 -> Product/2

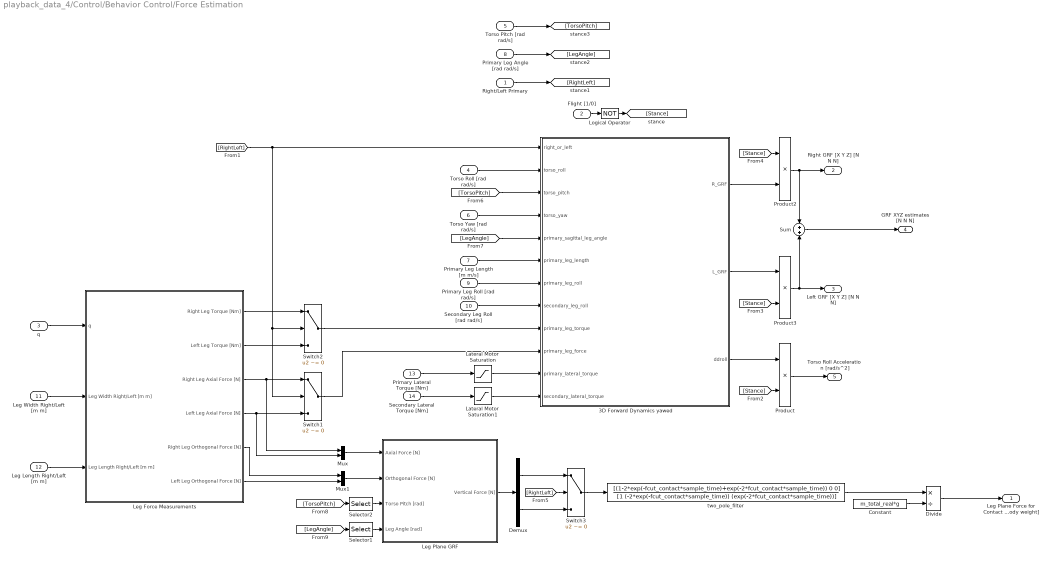
== system playback_data_4/Control/Behavior Control/Force Estimation ==
  Right/Left Primary : Inport
  Flight [1/0] : Inport  Port=2
  q : Inport  Port=3
  Torso Roll [rad rad/s] : Inport  Port=4
  Torso Pitch [rad rad/s] : Inport  Port=5
  Torso Yaw [rad rad/s] : Inport  Port=6
  Primary Leg Length [m m/s] : Inport  Port=7
  Primary Leg Angle [rad rad/s] : Inport  Port=8
  Primary Leg Roll [rad rad/s] : Inport  Port=9
  Secondary Leg Roll [rad rad/s] : Inport  Port=10
  Leg Width Right/Left [m m] : Inport  Port=11
  Leg Length Right/Left [m m] : Inport  Port=12
  Primary Lateral Torque [Nm] : Inport  Port=13
  Secondary Lateral Torque [Nm] : Inport  Port=14
  3D Forward Dynamics yawed : MATLAB Function  TreatAsAtomicUnit=on
  Constant : Constant  Value=m_total_real*g
  Demux : Demux  Outputs=2
  Divide : Product  Inputs=*/
  Lateral Motor Saturation : Saturate  UpperLimit=HIP_MTR_MAX_TORQUE  LowerLimit=-HIP_MTR_MAX_TORQUE
      settings: AttributesFormatString=Top: %<UpperLimit>\nBottom: %<LowerLimit>
  Lateral Motor Saturation1 : Saturate  UpperLimit=HIP_MTR_MAX_TORQUE  LowerLimit=-HIP_MTR_MAX_TORQUE
      settings: AttributesFormatString=Top: %<UpperLimit>\nBottom: %<LowerLimit>
  Leg Force Measurements : Subsystem
  Leg Plane GRF : Subsystem
  Logical Operator : Logic  Operator=NOT  AllPortsSameDT=off  OutDataTypeStr=boolean
  Mux : Mux  Inputs=2
  Mux1 : Mux  Inputs=2
  Product : Product
  Product2 : Product
  Product3 : Product
  Selector1 : Selector  InputPortWidth=2  Indices=[1]
  Selector2 : Selector  InputPortWidth=2  Indices=[1]
  Sum : Sum  Inputs=+|+
  Switch1 : Switch  Criteria=u2 ~= 0
  Switch2 : Switch  Criteria=u2 ~= 0
  Switch3 : Switch  Criteria=u2 ~= 0
  two_pole_filter : DiscreteTransferFcn  Numerator=[(1-2*exp(-fcut_contact*sample_time)+exp(-2*fcut_contact*sample_time)) 0 0]  Denominator=[1 (-2*exp(-fcut_contact*sample_time)) (exp(-2*fcut_contact*sample_time))]  SampleTime=sample_time
  Leg Plane Force for Contact Detection [body weight] : Outport
  Right GRF [X Y Z] [N N N] : Outport  Port=2
  Left GRF [X Y Z] [N N N] : Outport  Port=3
  GRF XYZ estimates [N N N] : Outport  Port=4  OutputWhenDisabled=reset  InitialOutput=[0 0 0 0 0 0]
  Torso Roll Acceleration [rad/s^2] : Outport  Port=5  OutputWhenDisabled=reset  InitialOutput=[0 0 0 0 0 0]
  wires:
  Lateral Motor Saturation1/1 -> 3D Forward Dynamics yawed/12(secondary_lateral_torque)
  Lateral Motor Saturation/1 -> 3D Forward Dynamics yawed/11(primary_lateral_torque)
  Secondary Lateral Torque [Nm]/1 -> Lateral Motor Saturation1/1
  Primary Lateral Torque [Nm]/1 -> Lateral Motor Saturation/1
  Selector2/1 -> Leg Plane GRF/3(Torso Pitch [rad])
  [TorsoPitch] -> Selector2/1
  Selector1/1 -> Leg Plane GRF/4(Leg Angle [rad])
  [LegAngle] -> Selector1/1
  Torso Pitch [rad rad/s]/1 -> [TorsoPitch]
  Primary Leg Angle [rad rad/s]/1 -> [LegAngle]
  Demux/2 -> Switch3/3
  Demux/1 -> Switch3/1
  Leg Plane GRF/1(Vertical Force [N]) -> Demux/1
  [RightLeft] -> Switch3/2
  Right/Left Primary/1 -> [RightLeft]
  Leg Force Measurements/6(Left Leg Orthogonal Force [N]) -> Mux1/2
  Leg Force Measurements/5(Right Leg Orthogonal Force [N]) -> Mux1/1
  Mux/1 -> Leg Plane GRF/1(Axial Force [N])
  Mux1/1 -> Leg Plane GRF/2(Orthogonal Force [N])
  Sum/1 -> GRF XYZ estimates [N N N]/1
  Leg Force Measurements/2(Left Leg Torque [Nm]) -> Switch2/3
  Leg Force Measurements/1(Right Leg Torque [Nm]) -> Switch2/1
  Switch2/1 -> 3D Forward Dynamics yawed/9(primary_leg_torque)
  Secondary Leg Roll [rad rad/s]/1 -> 3D Forward Dynamics yawed/8(secondary_leg_roll)
  Primary Leg Roll [rad rad/s]/1 -> 3D Forward Dynamics yawed/7(primary_leg_roll)
  [Stance] -> Product2/1
  [Stance] -> Product3/2
  Product2/1 -> Sum/1, Right GRF [X Y Z] [N N N]/1
  Product3/1 -> Sum/2, Left GRF [X Y Z] [N N N]/1
  Logical Operator/1 -> [Stance]
  Switch3/1 -> two_pole_filter/1
  Product/1 -> Torso Roll Acceleration [rad/s^2]/1
  [Stance] -> Product/2
  Flight [1/0]/1 -> Logical Operator/1
  [LegAngle] -> 3D Forward Dynamics yawed/5(primary_sagittal_leg_angle)
  Primary Leg Length [m m/s]/1 -> 3D Forward Dynamics yawed/6(primary_leg_length)
  Torso Yaw [rad rad/s]/1 -> 3D Forward Dynamics yawed/4(torso_yaw)
  Torso Roll [rad rad/s]/1 -> 3D Forward Dynamics yawed/2(torso_roll)
  [TorsoPitch] -> 3D Forward Dynamics yawed/3(torso_pitch)
  Switch1/1 -> 3D Forward Dynamics yawed/10(primary_leg_force)
  Leg Force Measurements/4(Left Leg Axial Force [N]) -> Mux/2, Switch1/3
  Leg Force Measurements/3(Right Leg Axial Force [N]) -> Switch1/1, Mux/1
  3D Forward Dynamics yawed/3(ddroll) -> Product/1
  3D Forward Dynamics yawed/2(L_GRF) -> Product3/1
  3D Forward Dynamics yawed/1(R_GRF) -> Product2/2
  Leg Length Right/Left [m m]/1 -> Leg Force Measurements/3(Leg Length Right/Left [m m])
  [RightLeft] -> Switch1/2, Switch2/2, 3D Forward Dynamics yawed/1(right_or_left)
  Constant/1 -> Divide/2
  two_pole_filter/1 -> Divide/1
  q/1 -> Leg Force Measurements/1(q)
  Leg Width Right/Left [m m]/1 -> Leg Force Measurements/2(Leg Width Right/Left [m m])
  Divide/1 -> Leg Plane Force for Contact Detection [body weight]/1

== system playback_data_4/Control/Behavior Control/L Leg Calculator ==
  Front [rad rad/s] : Inport
  Back [rad rad/s] : Inport  Port=2
  Constant : Constant  Value=d_ankle_to_foot-0.01
  Demux1 : Demux  Outputs=2
  Gain1 : Gain  Gain=2*l_seg
  Gain2 : Gain  Gain=l_seg
  Gain3 : Gain  Gain=-1
  Gain4 : Gain  Gain=0.5
  Gain5 : Gain  Gain=0.5
  Gain6 : Gain  Gain=2
  Mux1 : Mux  Inputs=2
  Product : Product  RndMeth=Zero
  Sum : Sum  Inputs=++|
  Sum4 : Sum  Inputs=+|+
  Sum5 : Sum  Inputs=+|-
  Trigonometric Function : Trigonometry  Operator=cos
  Trigonometric Function1 : Trigonometry
  "Leg Length [m m/s] " : Outport
  Leg Angle [rad rad/s] : Outport  Port=2
  Leg Splay [rad rad/s] : Outport  Port=3
  w [m] : Outport  Port=4
  wires:
  Gain5/1 -> Leg Angle [rad rad/s]/1
  Gain6/1 -> w [m]/1
  Gain4/1 -> Trigonometric Function1/1, Trigonometric Function/1
  Trigonometric Function/1 -> Gain1/1
  Gain1/1 -> Sum/2
  Trigonometric Function1/1 -> Gain2/1
  Product/1 -> Mux1/2
  Front [rad rad/s]/1 -> Sum5/2, Sum4/2
  Back [rad rad/s]/1 -> Sum4/1, Sum5/1
  Demux1/2 -> Gain3/1
  Gain3/1 -> Product/2
  Demux1/1 -> Gain4/1
  Gain2/1 -> Product/1, Gain6/1
  Sum5/1 -> Leg Splay [rad rad/s]/1, Demux1/1
  Mux1/1 -> "Leg Length [m m/s] "/1
  Sum4/1 -> Gain5/1
  Constant/1 -> Sum/1
  Sum/1 -> Mux1/1
